simulink model "Simulink_model"  (R2025b)
settings: Solver=FixedStepAuto  StartTime=0.0  StopTime=20  FixedStep=1e-3  RelTol=1e-3
values from neighbouring files (symbols this model uses):
  b = 0.05    [Data.m]
  g = 9.81    [Data.m]
  l = 0.25    [Data.m]
  m = 1    [Data.m]
  theta0_pt1 = deg2rad(theta0_deg_pt1)    [Data.m]
  theta0_pt2 = deg2rad(theta0_deg_pt2)    [Data.m]
  theta0dot_pt1 = deg2rad(theta0dot_deg_pt1)    [Data.m]
  theta0dot_pt2 = deg2rad(theta0dot_deg_pt2)    [Data.m]
settings Model: Creator=Enrico 2  LastModifiedBy=Enrico

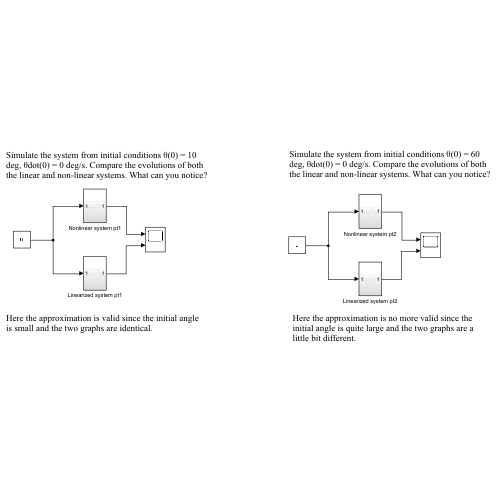
[thumbnail: Simulink's stored preview of the top-level diagram]
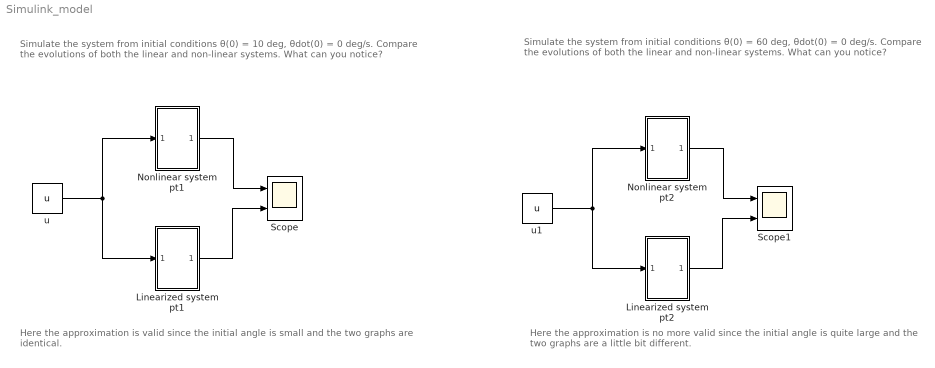
== system Simulink_model ==
  note: Simulate the system from initial conditions θ(0) = 10 deg, θdot(0) = 0 deg/s. Compare the evolutions of both the linear and non-linear systems. What can you notice?
  note: Simulate the system from initial conditions θ(0) = 60 deg, θdot(0) = 0 deg/s. Compare the evolutions of both the linear and non-linear systems. What can you notice?
  note: Here the approximation is valid since the initial angle is small and the two graphs are identical.
  note: Here the approximation is no more valid since the initial angle is quite large and the two graphs are a little bit different.
  Linearized system pt1 : Subsystem
  Linearized system pt2 : Subsystem
  Nonlinear system pt1 : Subsystem
  Nonlinear system pt2 : Subsystem
  Scope : Scope  NumInputPorts=2
      settings: ActiveDisplayYMinimum=-0.18240996565774259  ActiveDisplayYMaximum=0.2141932464057858
  Scope1 : Scope  NumInputPorts=2
      settings: ActiveDisplayYMinimum=-1.0944597939464551  ActiveDisplayYMaximum=1.2851594784347147
  u : Constant  Value=u
  u1 : Constant  Value=u
  wires:
  u/1 -> Linearized system pt1/1(In1), Nonlinear system pt1/1(In1)
  Nonlinear system pt1/1(Out1) -> Scope/1
  Linearized system pt1/1(Out1) -> Scope/2
  u1/1 -> Linearized system pt2/1(In1), Nonlinear system pt2/1(In1)
  Nonlinear system pt2/1(Out1) -> Scope1/1
  Linearized system pt2/1(Out1) -> Scope1/2

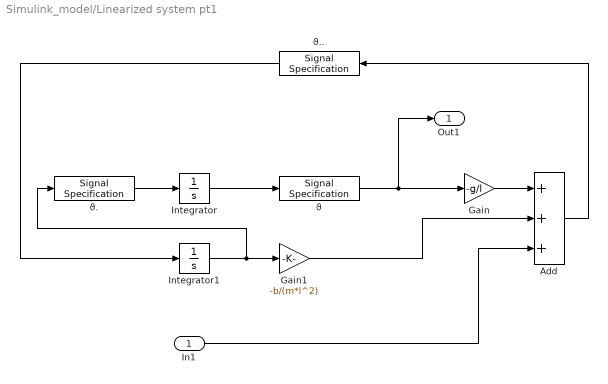
== system Simulink_model/Linearized system pt1 ==
  In1 : Inport
  Add : Sum  Inputs=+++
  Gain : Gain  Gain=-g/l
  Gain1 : Gain  Gain=-b/(m*l^2)
  Integrator : Integrator  InitialCondition=theta0_pt1
  Integrator1 : Integrator  InitialCondition=theta0dot_pt1
  ϑ : SignalSpecification  Unit=rad
  ϑ. : SignalSpecification  Unit=rad/sec
  ϑ.. : SignalSpecification  Unit=rad/sec^2
  Out1 : Outport
  wires:
  Integrator1/1 -> ϑ./1, Gain1/1
  Integrator/1 -> ϑ/1
  ϑ/1 -> Gain/1, Out1/1
  In1/1 -> Add/3
  Gain1/1 -> Add/2
  ϑ../1 -> Integrator1/1
  Gain/1 -> Add/1
  Add/1 -> ϑ../1
  ϑ./1 -> Integrator/1

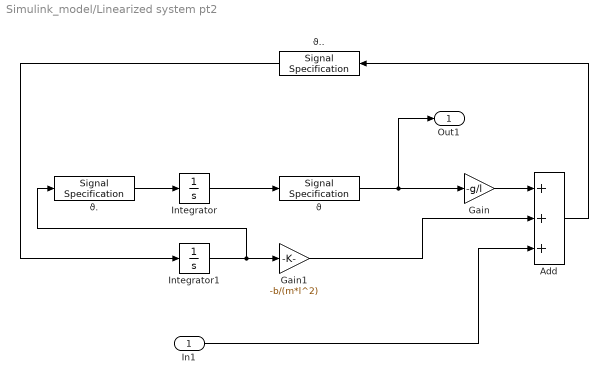
== system Simulink_model/Linearized system pt2 ==
  In1 : Inport
  Add : Sum  Inputs=+++
  Gain : Gain  Gain=-g/l
  Gain1 : Gain  Gain=-b/(m*l^2)
  Integrator : Integrator  InitialCondition=theta0_pt2
  Integrator1 : Integrator  InitialCondition=theta0dot_pt2
  ϑ : SignalSpecification  Unit=rad
  ϑ. : SignalSpecification  Unit=rad/sec
  ϑ.. : SignalSpecification  Unit=rad/sec^2
  Out1 : Outport
  wires:
  Integrator1/1 -> ϑ./1, Gain1/1
  Integrator/1 -> ϑ/1
  ϑ/1 -> Gain/1, Out1/1
  In1/1 -> Add/3
  Gain1/1 -> Add/2
  ϑ../1 -> Integrator1/1
  Gain/1 -> Add/1
  Add/1 -> ϑ../1
  ϑ./1 -> Integrator/1

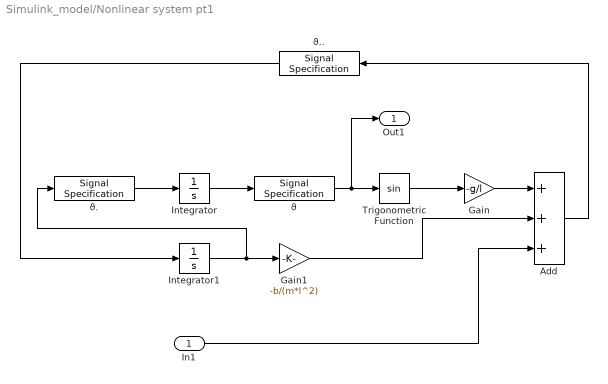
== system Simulink_model/Nonlinear system pt1 ==
  In1 : Inport
  Add : Sum  Inputs=+++
  Gain : Gain  Gain=-g/l
  Gain1 : Gain  Gain=-b/(m*l^2)
  Integrator : Integrator  InitialCondition=theta0_pt1
  Integrator1 : Integrator  InitialCondition=theta0dot_pt1
  Trigonometric Function : Trigonometry
  ϑ : SignalSpecification  Unit=rad
  ϑ. : SignalSpecification  Unit=rad/sec
  ϑ.. : SignalSpecification  Unit=rad/sec^2
  Out1 : Outport
  wires:
  Integrator1/1 -> ϑ./1, Gain1/1
  Integrator/1 -> ϑ/1
  ϑ/1 -> Out1/1, Trigonometric Function/1
  In1/1 -> Add/3
  Gain1/1 -> Add/2
  ϑ../1 -> Integrator1/1
  Gain/1 -> Add/1
  Add/1 -> ϑ../1
  ϑ./1 -> Integrator/1
  Trigonometric Function/1 -> Gain/1

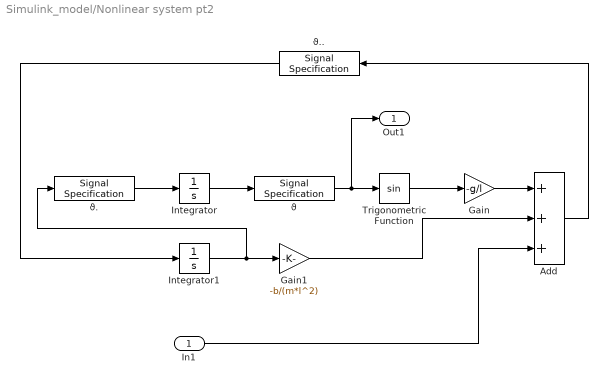
== system Simulink_model/Nonlinear system pt2 ==
  In1 : Inport
  Add : Sum  Inputs=+++
  Gain : Gain  Gain=-g/l
  Gain1 : Gain  Gain=-b/(m*l^2)
  Integrator : Integrator  InitialCondition=theta0_pt2
  Integrator1 : Integrator  InitialCondition=theta0dot_pt2
  Trigonometric Function : Trigonometry
  ϑ : SignalSpecification  Unit=rad
  ϑ. : SignalSpecification  Unit=rad/sec
  ϑ.. : SignalSpecification  Unit=rad/sec^2
  Out1 : Outport
  wires:
  Integrator1/1 -> ϑ./1, Gain1/1
  Integrator/1 -> ϑ/1
  ϑ/1 -> Out1/1, Trigonometric Function/1
  In1/1 -> Add/3
  Gain1/1 -> Add/2
  ϑ../1 -> Integrator1/1
  Gain/1 -> Add/1
  Add/1 -> ϑ../1
  ϑ./1 -> Integrator/1
  Trigonometric Function/1 -> Gain/1
